simulink model "variant_subsystem"  (R2020b)
settings: Solver=VariableStepAuto  StartTime=0.0  StopTime=10.0  RelTol=1e-3
settings Model: Creator=Training  LastModifiedBy=Training

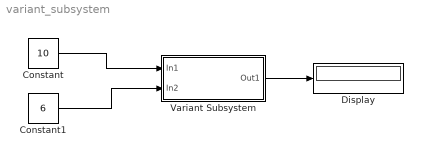
== system variant_subsystem ==
  Constant : Constant  Value=10
  Constant1 : Constant  Value=6
  Display : Display
  Variant Subsystem : Subsystem  Variant=on
  wires:
  Constant/1 -> Variant Subsystem/1(In1)
  Constant1/1 -> Variant Subsystem/2(In2)
  Variant Subsystem/1(Out1) -> Display/1

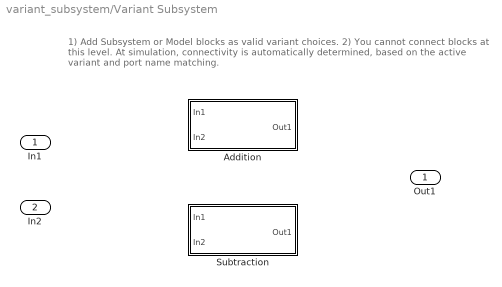
== system variant_subsystem/Variant Subsystem ==
  note: 1) Add Subsystem or Model blocks as valid variant choices.
      | 2) You cannot connect blocks at this level. At simulation, connectivity is automatically
      | determined, based on the active variant and port name matching.
  In1 : Inport
  In2 : Inport  Port=2
  Addition : Subsystem  VariantControl=Choice_1
  Subtraction : Subsystem  VariantControl=Choice_2
  Out1 : Outport

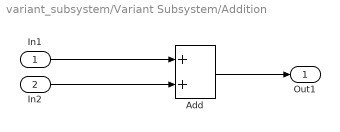
== system variant_subsystem/Variant Subsystem/Addition ==
  In1 : Inport
  In2 : Inport  Port=2
  Add : Sum
  Out1 : Outport
  wires:
  In1/1 -> Add/1
  In2/1 -> Add/2
  Add/1 -> Out1/1

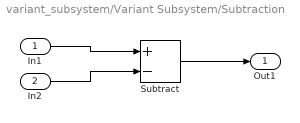
== system variant_subsystem/Variant Subsystem/Subtraction ==
  In1 : Inport
  In2 : Inport  Port=2
  Subtract : Sum  Inputs=+-
  Out1 : Outport
  wires:
  In1/1 -> Subtract/1
  In2/1 -> Subtract/2
  Subtract/1 -> Out1/1
